simulink model "FG_Simulator"  (R2017b)
settings: Solver=VariableStepAuto  StartTime=0  StopTime=10  FixedStep=0.0005  EnableMultiTasking=on
InitFcn:
  | isSim = 1;
  | PreFunctions.CustomInitFcn;
  | PreFunctions.simulationInitFcn
values from neighbouring files (symbols this model uses):
  s = min(s_unsat,1.05)    [FG_Controller_v1.m]    (also in FG_Controller_v2.m)
undefined symbols (not defined in the file or in its folder): DiagnosticCodes, motorPositions, motorVelocities, pelvisPosition, pelvisVelocity, UserParams, X, Y, Z
libraries: sm_lib x12, CassieLibrary x3, nesl_utility x1, FG_Controller_Library x1
settings Model: Creator=case  LastModifiedBy=Sunny
settings SolverCC: ZeroCrossControl=DisableAll  InsertRTBMode=Always
settings DataIOCC: SaveOutput=off  SignalLogging=off  DSMLogging=off  SaveTime=off
settings OptimizationCC: DefaultParameterBehavior=Inlined  UseFloatMulNetSlope=on  InlineInvariantSignals=on  EfficientFloat2IntCast=on  LifeSpan=inf  SimCompilerOptimization=on  AccelVerboseBuild=on
settings DebuggingCC: ReadBeforeWriteMsg=DisableAll  WriteAfterWriteMsg=DisableAll  WriteAfterReadMsg=DisableAll  ParameterUnderflowMsg=error  ParameterTunabilityLossMsg=error  UniqueDataStoreMsg=error  AllowSymbolicDim=off  StrictBusMsg=ErrorOnBusTreatedAsVector  SFUnexpectedBacktrackingDiag=warning  SFNoUnconditionalDefaultTransitionDiag=warning  SFExecutionAtInitializationDiag=none
settings HardwareCC: TargetBitPerPointer=64  TargetBitPerSizeT=64  TargetBitPerPtrDiffT=64  TargetLongLongMode=on  TargetIntDivRoundTo=Zero  TargetEndianess=LittleEndian  TargetWordSize=64  TargetHWDeviceType=MATLAB Host  ProdEqTarget=off
settings ModelReferenceCC: EnableParallelModelReferenceBuilds=on  ModelReferenceNumInstancesAllowed=Zero  ModelReferenceMinAlgLoopOccurrences=on  PropagateSignalLabelsOutOfModel=off
settings SFSimCC: SimUserIncludeDirs=D:\Graduate\robots\Cassie\GitHub\Cassie_Controller_V3_Yukai\Controllers\Flatground\utils\funcs\kin
settings SFSimCC: SimUserSources=|
  | ComPosition_src.c
  | ComVelocity_src.c
  | J_LeftToeBottomBack_src.c
  | J_LeftToeBottomFront_src.c
  | J_LeftToeBottom_src.c
  | J_LeftToeJoint_src.c
  | J_RightToeBottomBack_src.c
  | J_RightToeBottomFront_src.c
  | J_RightToeBottom_src.c
  | J_RightToeJoint_src.c
  | LeftToeBottomBack_src.c
  | LeftToeBottomFront_src.c
  | LeftToeBottom_src.c
  | LeftToeJoint_src.c
  | RightToeBottomBack_src.c
  | RightToeBottomFront_src.c
  | RightToeBottom_src.c
  | RightToeJoint_src.c
settings RTWCC: Description=Generic Real-Time Target  RTWUseSimCustomCode=on  CustomInclude=D:\Graduate\robots\Cassie\GitHub\Cassie_Controller_V3_Yukai\Controllers\Flatground\utils\funcs\kin  BuildConfiguration=Faster Runs  CheckMdlBeforeBuild=Warning
settings RTWCC: CustomSource=|
  | ComPosition_src.c
  | ComVelocity_src.c
  | J_LeftToeBottomBack_src.c
  | J_LeftToeBottomFront_src.c
  | J_LeftToeBottom_src.c
  | J_LeftToeJoint_src.c
  | J_RightToeBottomBack_src.c
  | J_RightToeBottomFront_src.c
  | J_RightToeBottom_src.c
  | J_RightToeJoint_src.c
  | LeftToeBottomBack_src.c
  | LeftToeBottomFront_src.c
  | LeftToeBottom_src.c
  | LeftToeJoint_src.c
  | RightToeBottomBack_src.c
  | RightToeBottomFront_src.c
  | RightToeBottom_src.c
  | RightToeJoint_src.c
settings CodeAppCC: GenerateComments=off  SimulinkBlockComments=off
settings GRTTargetCC: MatFileLogging=off  MultiInstanceERTCode=on  CodeInterfacePackaging=Reusable function  SupportNonFinite=off  GenerateAllocFcn=on
settings ConfigComp: CovMetricSettings=dw  CovHtmlReporting=on  CovSaveCumulativeToWorkspaceVar=on  CovSaveSingleToWorkspaceVar=on  CovExternalEMLEnable=off
settings SimscapeCC: SimscapeNormalizeSystem=off
settings DiagnosticsConfigSet: SimMechanicsRigidlyBoundBlock=warning
settings ExplorerConfigSet: InternalSimMechanicsExplorerSettings="<ExplorerConfiguration><canonicalview>default</canonicalview><AnimationSetting><BasePlaybackSpeed>1.0</BasePlaybackSpeed><PlaybackSpeedFactor>1.0</PlaybackSpeedFactor></AnimationSetting><TilePanel><TileInfo><Tiles Columns=\"1\" Count=\"1\" Rows=\"1\"><Column Weight=\"1\"/><Row Weight=\"1\"/><Tile Height=\"1\" Width=\"1\" X=\"0\" Y=\"0\"/></Tiles></TileInfo><SceneInfo><SceneViewer><BGColor><R>0.60000002384185791</R><G>0.60000002384185791</G><B>0.60000002384185791</B></BGColor><Camera><DoPerspective>on</DoPerspective><Position><X>1.49424103443841916</X><Y>-1.5003618867302666</Y><Z>-0.448846928440659099</Z></Position><Center><X>-0.00575896556158084216</X><Y>-0.000361886730266602896</Y><Z>-0.948846928440659099</Z></Center><Up><X>0</X><Y>0</Y><Z>1</Z></Up><ViewLimDist>1</ViewLimDist><YLim>0.466307658154998583</YLim><XLim>2.07568807125632082</XLim></Camera></SceneViewer></SceneInfo></TilePanel><MechEditorPanel><Cameras><Camera><Id>Camera1</Id><Value><Name>Tracking Camera</Name><NativeCamera><PositionTrackingFeature>Cassie.Cassie_Simulation.World.Tracking_Camera.F</PositionTrackingFeature><CenterTrackingFeature>Cassie.Cassie_Simulation.World.Tracking_Camera_Target.F</CenterTrackingFeature><UpVectorTrackingFeature>Cassie.Cassie_Simulation.World.Tracking_Camera_Target.F</UpVectorTrackingFeature><CenterTrackingOrigin>on</CenterTrackingOrigin><UpVectorTrackingDirection>+Z</UpVectorTrackingDirection></NativeCamera></Value></Camera><Camera><Id>Camera2</Id><Value><Name>Fixed Camera</Name><NativeCamera><PositionTrackingFeature>Cassie.Cassie_Simulation.World.Fixed_Camera.F</PositionTrackingFeature><CenterTrackingFeature>Cassie.Cassie_Simulation.World.Fixed_Camera_Target.F</CenterTrackingFeature><UpVectorTrackingFeature>Cassie.Cassie_Simulation.World.Fixed_Camera_Target.F</UpVectorTrackingFeature><CenterTrackingOrigin>on</CenterTrackingOrigin><UpVectorTrackingDirection>+Z</UpVectorTrackingDirection></NativeCamera></Value></Camera></Cameras><GfxPanelCameraMap><MapElement CameraMLId=\"Camera1\" GfxPanelIndex=\"0\"/></GfxPanelCameraMap><VideoCreator><PlaybackSpeedRatio>1.0</PlaybackSpeedRatio><FrameRate>30</FrameRate><VideoFormat>Motion JPEG AVI</VideoFormat><FrameSize>auto</FrameSize></VideoCreator></MechEditorPanel></ExplorerConfiguration>"

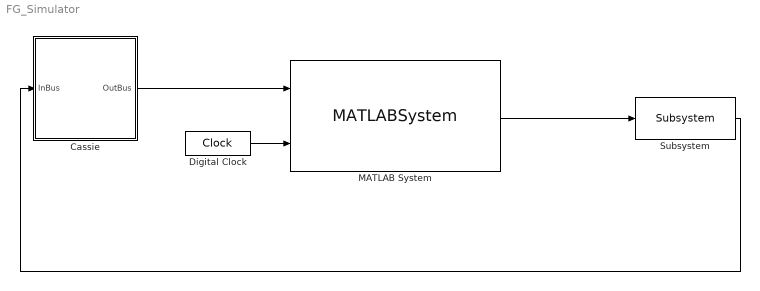
== system FG_Simulator ==
  Cassie : Subsystem  AncestorBlock=CassieLibrary/Simulation/Cassie  InitFcn=|  StartFcn=|  StopFcn=|
      InitFcn=|
      | % Start clock at initialization (used for computing real time performance)
      | initTime = tic;
      | 
      | % Import bus definitions
      | CassieModule.importBuses;
      StartFcn=|
      | % Store build time
      | buildTime = toc(initTime);
      StopFcn=|
      | % Store computation time
      | computationTime = toc(initTime) - buildTime;
      | 
      | % Get simulation time
      | simulationTime = get_param(bdroot, 'SimulationTime');
      | 
      | % Compute real time performance
      | percentRealTime = 100*simulationTime/computationTime;
      | 
      | % Display
      | fprintf('Build time: %0.2f seconds \n', buildTime);
      | fprintf('Simulation time: %0.2f seconds \n', simulationTime);
      | fprintf('Computation time: %0.2f seconds \n', computationTime);
      | fprintf('Performance: %0.2f%% real time \n', percentRealTime);
      mask Display: image('Cassie.png');
  Digital Clock : DigitalClock  SampleTime=UserParams.SampleTime
  MATLAB System : MATLABSystem  System=RemoteSpoofer  SimulateUsing=Code generation
      mask Type: RemoteSpoofer
      mask Display:
      | disp('RemoteSpoofer');
      | port_label('input',1,'cassieOutputs');
      | port_label('input',2,'t');
      | port_label('output',1,'cassieOutputs');
  Subsystem : FG_Controller_Library/Subsystem
  wires:
  Cassie/1(OutBus) -> MATLAB System/1
  Digital Clock/1 -> MATLAB System/2
  MATLAB System/1 -> Subsystem/1
  Subsystem/1 -> Cassie/1(InBus)

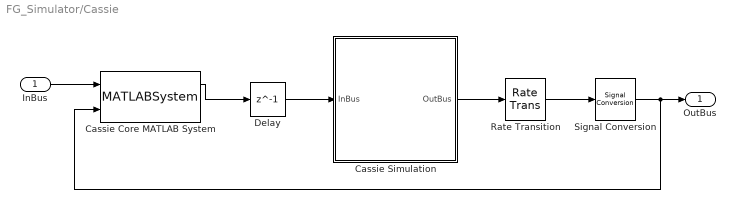
== system FG_Simulator/Cassie ==
  InBus : Inport  OutDataTypeStr=Bus: CassieUserInBus
  Cassie Core MATLAB System : MATLABSystem  System=CassieCoreSim  SimulateUsing=Code generation
      mask Type: CassieCoreSim
      mask Display: disp('CassieCoreSim');
  Cassie Simulation : Subsystem  AncestorBlock=CassieLibrary/Simulation/Cassie Simulation
      mask Display: image('Cassie.png');
  Delay : Delay  DelayLength=1
  Rate Transition : RateTransition  OutPortSampleTime=0.0005
  Signal Conversion : SignalConversion  ConversionOutput=Nonvirtual bus  OutDataTypeStr=Bus: CassieOutBus  OverrideOpt=off
  OutBus : Outport  OutDataTypeStr=Bus: CassieOutBus
  wires:
  Signal Conversion/1 -> OutBus/1, Cassie Core MATLAB System/2
  Cassie Simulation/1(OutBus) -> Rate Transition/1
  Rate Transition/1 -> Signal Conversion/1
  Delay/1 -> Cassie Simulation/1(InBus)
  Cassie Core MATLAB System/1 -> Delay/1
  InBus/1 -> Cassie Core MATLAB System/1

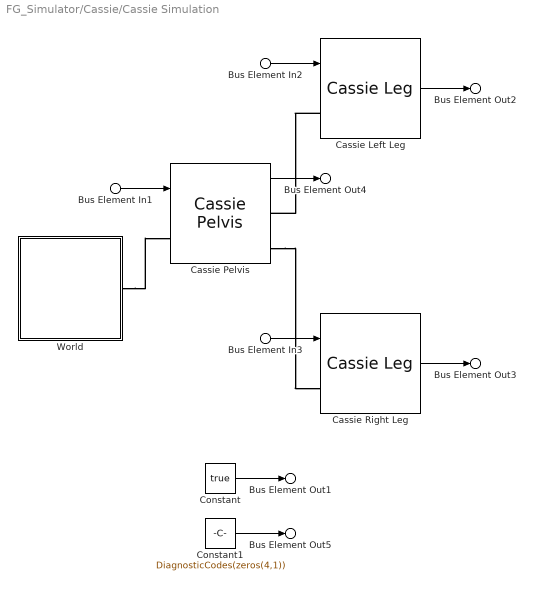
== system FG_Simulator/Cassie/Cassie Simulation ==
  Bus Element In2 : Inport  PortName=InBus  Element=leftLeg
  Bus Element In3 : Inport  PortName=InBus  Element=rightLeg
  Bus Element In1 : Inport  PortName=InBus  Element=pelvis
  Cassie Left Leg : CassieLibrary/Simulation/Cassie Leg  config=Left  motorPositions=motorPositions(1:5)  motorVelocities=motorVelocities(1:5)
  Cassie Pelvis : CassieLibrary/Simulation/Cassie Pelvis  SystemSampleTime=-1
  Cassie Right Leg : CassieLibrary/Simulation/Cassie Leg  config=Right  motorPositions=motorPositions(6:10)  motorVelocities=motorVelocities(6:10)
  Constant : Constant  Value=true
  Constant1 : Constant  Value=DiagnosticCodes(zeros(4,1))
  World : Subsystem  AncestorBlock=ComponentLibrary/Simulation/World
  Bus Element Out4 : Outport  PortName=OutBus  Element=pelvis
  Bus Element Out2 : Outport  PortName=OutBus  Element=leftLeg
  Bus Element Out3 : Outport  PortName=OutBus  Element=rightLeg
  Bus Element Out1 : Outport  PortName=OutBus  Element=isCalibrated
  Bus Element Out5 : Outport  PortName=OutBus  Element=messages
  wires:
  Constant1/1 -> Bus Element Out5/1
  Constant/1 -> Bus Element Out1/1
  Bus Element In1/1 -> Cassie Pelvis/1
  Cassie Right Leg/1 -> Bus Element Out3/1
  Bus Element In2/1 -> Cassie Left Leg/1
  Cassie Left Leg/1 -> Bus Element Out2/1
  Bus Element In3/1 -> Cassie Right Leg/1
  Cassie Pelvis/1 -> Bus Element Out4/1
  connections:
  World/RConn1 -- Cassie Pelvis/LConn1
  Cassie Left Leg/LConn1 -- Cassie Pelvis/RConn1
  Cassie Pelvis/RConn2 -- Cassie Right Leg/LConn1

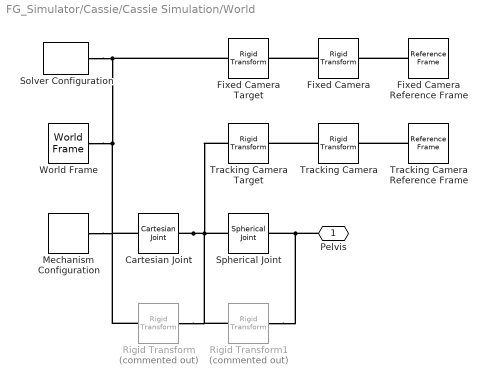
== system FG_Simulator/Cassie/Cassie Simulation/World ==
  Cartesian Joint : sm_lib/Joints/Cartesian Joint  SenseConstraintForce=off  SenseConstraintForceX=off  SenseConstraintForceY=off  SenseConstraintForceZ=off  SenseConstraintTorque=off  SenseConstraintTorqueX=off  SenseConstraintTorqueY=off  SenseConstraintTorqueZ=off  SenseTotalForce=off  SenseTotalForceX=off  SenseTotalForceY=off  SenseTotalForceZ=off  SenseTotalTorque=off  SenseTotalTorqueX=off  SenseTotalTorqueY=off  SenseTotalTorqueZ=off  CompositeWrenchDir=FollowerOnBase  CompositeWrenchFrame=BaseFrame  PxEquilibriumPosition=0  PxEquilibriumPositionUnits=m  PxSpringStiffness=0  PxSpringStiffnessUnits=N/m  PxDampingCoefficient=0  PxDampingCoefficientUnits=N/(m/s)  PxTorqueActuationMode=NoTorque  PxMotionActuationMode=ComputedMotion  PxSensePosition=off  PxSenseVelocity=off  PxSenseAcceleration=off  PxSenseTorqueForce=off  PxPositionTargetSpecify=on  PxPositionTargetPriority=High  PxPositionTargetValue=pelvisPosition(1)  PxPositionTargetValueUnits=m  PxVelocityTargetSpecify=on  PxVelocityTargetPriority=High  PxVelocityTargetValue=pelvisVelocity(1)  PxVelocityTargetValueUnits=m/s  PyEquilibriumPosition=0  PyEquilibriumPositionUnits=m  PySpringStiffness=0  PySpringStiffnessUnits=N/m  PyDampingCoefficient=0  PyDampingCoefficientUnits=N/(m/s)  PyTorqueActuationMode=NoTorque  PyMotionActuationMode=ComputedMotion  PySensePosition=off  PySenseVelocity=off  PySenseAcceleration=off  PySenseTorqueForce=off  PyPositionTargetSpecify=on  PyPositionTargetPriority=High  PyPositionTargetValue=pelvisPosition(2)  PyPositionTargetValueUnits=m  PyVelocityTargetSpecify=on  PyVelocityTargetPriority=High  PyVelocityTargetValue=pelvisVelocity(2)  PyVelocityTargetValueUnits=m/s  PzEquilibriumPosition=0  PzEquilibriumPositionUnits=m  PzSpringStiffness=0  PzSpringStiffnessUnits=N/m  PzDampingCoefficient=0  PzDampingCoefficientUnits=N/(m/s)  PzTorqueActuationMode=NoTorque  PzMotionActuationMode=ComputedMotion  PzSensePosition=off  PzSenseVelocity=off  PzSenseAcceleration=off  PzSenseTorqueForce=off  PzPositionTargetSpecify=on  PzPositionTargetPriority=High  PzPositionTargetValue=pelvisPosition(3)  PzPositionTargetValueUnits=m  PzVelocityTargetSpecify=on  PzVelocityTargetPriority=High  PzVelocityTargetValue=pelvisVelocity(3)  PzVelocityTargetValueUnits=m/s
  Fixed Camera : sm_lib/Frames and Transforms/Rigid Transform  TranslationMethod=Cartesian  TranslationStandardOffset=0  TranslationLengthUnit=m  TranslationStandardAxis=+Z  TranslationCartesianOffset=[1.5 -1.5 0.5]  TranslationROffset=0  TranslationROffsetUnits=m  TranslationZOffset=0  TranslationZOffsetUnits=m  TranslationThetaOffset=0  TranslationThetaOffsetUnits=deg  RotationMethod=None  RotationAngleUnits=deg  RotationStandardAxis=+Z  RotationAngle=0.0  RotationArbitraryAxis=[0 0 1]  FollAlignAxisA=+X  BaseAlignAxisA=+Y  FollAlignAxisB=+Y  BaseAlignAxisB=+Z  RotationSequenceAxes=FollowerAxes  RotationSequence=XYX  RotationSequenceAngles=[0 0 0]  RotationSequenceAnglesUnits=deg  RotationMatrix=[1 0 0; 0 1 0; 0 0 1]
  Fixed Camera Target : sm_lib/Frames and Transforms/Rigid Transform  TranslationMethod=Cartesian  TranslationStandardOffset=0  TranslationLengthUnit=m  TranslationStandardAxis=+Z  TranslationCartesianOffset=[0 0 0.5]  TranslationROffset=0  TranslationROffsetUnits=m  TranslationZOffset=0  TranslationZOffsetUnits=m  TranslationThetaOffset=0  TranslationThetaOffsetUnits=deg  RotationMethod=None  RotationAngleUnits=deg  RotationStandardAxis=+Z  RotationAngle=0.0  RotationArbitraryAxis=[0 0 1]  FollAlignAxisA=+X  BaseAlignAxisA=+Y  FollAlignAxisB=+Y  BaseAlignAxisB=+Z  RotationSequenceAxes=FollowerAxes  RotationSequence=XYX  RotationSequenceAngles=[0 0 0]  RotationSequenceAnglesUnits=deg  RotationMatrix=[1 0 0; 0 1 0; 0 0 1]
  Fixed Camera Reference Frame : sm_lib/Frames and Transforms/Reference Frame
  Mechanism Configuration : sm_lib/Utilities/Mechanism Configuration  UniformGravity=Constant  GravityVector=[0 0 -9.80665]  GravityUnits=m/s^2  LinearizationDelta=0.001
  Rigid Transform : sm_lib/Frames and Transforms/Rigid Transform  Commented=on  TranslationMethod=Cartesian  TranslationStandardOffset=0  TranslationLengthUnit=m  TranslationStandardAxis=+Z  TranslationCartesianOffset=pelvisPosition  TranslationROffset=0  TranslationROffsetUnits=m  TranslationZOffset=0  TranslationZOffsetUnits=m  TranslationThetaOffset=0  TranslationThetaOffsetUnits=deg  RotationMethod=None  RotationAngleUnits=deg  RotationStandardAxis=+Z  RotationAngle=0.0  RotationArbitraryAxis=[0 0 1]  FollAlignAxisA=+X  BaseAlignAxisA=+Y  FollAlignAxisB=+Y  BaseAlignAxisB=+Z  RotationSequenceAxes=FollowerAxes  RotationSequence=XYX  RotationSequenceAngles=[0 0 0]  RotationSequenceAnglesUnits=deg  RotationMatrix=[1 0 0; 0 1 0; 0 0 1]
  Rigid Transform1 : sm_lib/Frames and Transforms/Rigid Transform  Commented=on  TranslationMethod=None  TranslationStandardOffset=0  TranslationLengthUnit=m  TranslationStandardAxis=+Z  TranslationCartesianOffset=[0 0 0]  TranslationROffset=0  TranslationROffsetUnits=m  TranslationZOffset=0  TranslationZOffsetUnits=m  TranslationThetaOffset=0  TranslationThetaOffsetUnits=deg  RotationMethod=RotationMatrix  RotationAngleUnits=deg  RotationStandardAxis=+Z  RotationAngle=0.0  RotationArbitraryAxis=[0 0 1]  FollAlignAxisA=+X  BaseAlignAxisA=+Y  FollAlignAxisB=+Y  BaseAlignAxisB=+Z  RotationSequenceAxes=FollowerAxes  RotationSequence=XYX  RotationSequenceAngles=[0 0 0]  RotationSequenceAnglesUnits=deg  RotationMatrix=pelvisRotation
  Solver Configuration : nesl_utility/Solver Configuration  PhysicalDomain=network_engine_domain  SubClassName=solver  LeftPortType=input  RightPortType=generic  Accelerate=off  Tones=[]  Harmonics=[]  SimulateNoise=off  Profile=off  UseLocalSampling=off  EnableSwitchedLinearOptims=on  FrequencyDomain=off  UseCCode=off  RelTol=0.001  AbsTol=1e-06  MinStep=1e-09  ToWorkspace=off  RevertToSquareIcSolve=off  NumHomotopyIterations=100  PhasorMode=off  PhasorModeNumHarmonics=1  DoDC=off  ResidualTolerance=1e-09  UseLocalSolver=off  LocalSolverChoice=NE_BACKWARD_EULER_ADVANCER  LocalSolverSampleTime=0.001  DoFixedCost=off  MaxNonlinIter=3  MaxModeIter=2  LinearAlgebra=Sparse  DelaysMemoryBudget=1024  AutomaticFiltering=on  FilteringTimeConstant=0.001
  Spherical Joint : sm_lib/Joints/Spherical Joint  SenseConstraintForce=off  SenseConstraintForceX=off  SenseConstraintForceY=off  SenseConstraintForceZ=off  SenseConstraintTorque=off  SenseConstraintTorqueX=off  SenseConstraintTorqueY=off  SenseConstraintTorqueZ=off  SenseTotalForce=off  SenseTotalForceX=off  SenseTotalForceY=off  SenseTotalForceZ=off  SenseTotalTorque=off  SenseTotalTorqueX=off  SenseTotalTorqueY=off  SenseTotalTorqueZ=off  CompositeWrenchDir=FollowerOnBase  CompositeWrenchFrame=BaseFrame  DefPosRotationMethod=None  DefPosRotationAngleUnits=deg  DefPosRotationStandardAxis=+Z  DefPosRotationAngle=0.0  DefPosRotationArbitraryAxis=[0 0 1]  DefPosFollAlignAxisA=+X  DefPosBaseAlignAxisA=+Y  DefPosFollAlignAxisB=+Y  DefPosBaseAlignAxisB=+Z  DefPosRotationSequenceAxes=FollowerAxes  DefPosRotationSequence=XYX  DefPosRotationSequenceAngles=[0 0 0]  DefPosRotationSequenceAnglesUnits=deg  DefPosRotationMatrix=[1 0 0; 0 1 0; 0 0 1]  EqPosRotationMethod=None  EqPosRotationAngleUnits=deg  EqPosRotationStandardAxis=+Z  EqPosRotationAngle=0.0  EqPosRotationArbitraryAxis=[0 0 1]  EqPosFollAlignAxisA=+X  EqPosBaseAlignAxisA=+Y  EqPosFollAlignAxisB=+Y  EqPosBaseAlignAxisB=+Z  EqPosRotationSequenceAxes=FollowerAxes  EqPosRotationSequence=XYX  EqPosRotationSequenceAngles=[0 0 0]  EqPosRotationSequenceAnglesUnits=deg  EqPosRotationMatrix=[1 0 0; 0 1 0; 0 0 1]  SpringStiffness=0  SpringStiffnessUnits=N*m/deg  DampingCoefficient=0  DampingCoefficientUnits=N*m/(deg/s)  ActuateTorqueX=off  ActuateTorqueY=off  ActuateTorqueZ=off  ActuateTorque=off  TorqueActuationMode=NoTorque  MotionActuationMode=ComputedMotion  ActuationFrame=BaseFrame  SensePosition=off  SenseVelocityX=off  SenseVelocityY=off  SenseVelocityZ=off  SenseVelocity=off  SenseAccelerationX=off  SenseAccelerationY=off  SenseAccelerationZ=off  SenseAcceleration=off  SenseTorqueX=off  SenseTorqueY=off  SenseTorqueZ=off  SenseTorqueForce=off  SensingFrame=BaseFrame  PositionTargetRotationMethod=RotationMatrix  PositionTargetRotationAngleUnits=deg  PositionTargetRotationStandardAxis=+Z  PositionTargetRotationAngle=0.0  PositionTargetRotationArbitraryAxis=[0 0 1]  PositionTargetFollAlignAxisA=+X  PositionTargetBaseAlignAxisA=+Y  PositionTargetFollAlignAxisB=+Y  PositionTargetBaseAlignAxisB=+Z  PositionTargetRotationSequenceAxes=FollowerAxes  PositionTargetRotationSequence=XYX  PositionTargetRotationSequenceAngles=[0 0 0]  PositionTargetRotationSequenceAnglesUnits=deg  PositionTargetRotationMatrix=pelvisRotation  PositionTargetSpecify=on  PositionTargetPriority=High  VelocityTargetValue=pelvisAngularVelocity  VelocityTargetValueUnits=rad/s  VelocityTargetSpecify=on  VelocityTargetPriority=High  VelocityTargetInFollowerFrame=on
  Tracking Camera : sm_lib/Frames and Transforms/Rigid Transform  TranslationMethod=Cartesian  TranslationStandardOffset=0  TranslationLengthUnit=m  TranslationStandardAxis=+Z  TranslationCartesianOffset=[1.5 -1.5 0.5]  TranslationROffset=0  TranslationROffsetUnits=m  TranslationZOffset=0  TranslationZOffsetUnits=m  TranslationThetaOffset=0  TranslationThetaOffsetUnits=deg  RotationMethod=None  RotationAngleUnits=deg  RotationStandardAxis=+Z  RotationAngle=0.0  RotationArbitraryAxis=[0 0 1]  FollAlignAxisA=+X  BaseAlignAxisA=+Y  FollAlignAxisB=+Y  BaseAlignAxisB=+Z  RotationSequenceAxes=FollowerAxes  RotationSequence=XYX  RotationSequenceAngles=[0 0 0]  RotationSequenceAnglesUnits=deg  RotationMatrix=[1 0 0; 0 1 0; 0 0 1]
  Tracking Camera Target : sm_lib/Frames and Transforms/Rigid Transform  TranslationMethod=Cartesian  TranslationStandardOffset=0  TranslationLengthUnit=m  TranslationStandardAxis=+Z  TranslationCartesianOffset=[0 0 -0.5]  TranslationROffset=0  TranslationROffsetUnits=m  TranslationZOffset=0  TranslationZOffsetUnits=m  TranslationThetaOffset=0  TranslationThetaOffsetUnits=deg  RotationMethod=None  RotationAngleUnits=deg  RotationStandardAxis=+Z  RotationAngle=0.0  RotationArbitraryAxis=[0 0 1]  FollAlignAxisA=+X  BaseAlignAxisA=+Y  FollAlignAxisB=+Y  BaseAlignAxisB=+Z  RotationSequenceAxes=FollowerAxes  RotationSequence=XYX  RotationSequenceAngles=[0 0 0]  RotationSequenceAnglesUnits=deg  RotationMatrix=[1 0 0; 0 1 0; 0 0 1]
  Tracking Camera Reference Frame : sm_lib/Frames and Transforms/Reference Frame
  World Frame : sm_lib/Frames and Transforms/World Frame
  Pelvis : PMIOPort  Port=1  Side=Right
  connections:
  Fixed Camera/LConn1 -- Fixed Camera Target/RConn1
  Fixed Camera Reference Frame/RConn1 -- Fixed Camera/RConn1
  Tracking Camera/LConn1 -- Tracking Camera Target/RConn1
  Tracking Camera Reference Frame/RConn1 -- Tracking Camera/RConn1
  Fixed Camera Target/LConn1 -- Solver Configuration/RConn1 -- Rigid Transform/LConn1 -- Cartesian Joint/LConn1 -- Mechanism Configuration/RConn1 -- World Frame/RConn1
  Pelvis/RConn1 -- Rigid Transform1/RConn1 -- Spherical Joint/RConn1
  Cartesian Joint/RConn1 -- Rigid Transform/RConn1 -- Rigid Transform1/LConn1 -- Tracking Camera Target/LConn1 -- Spherical Joint/LConn1
